simulink model "FAST"  (R2017b)
settings: Solver=FixedStepAuto  StartTime=0.0  StopTime=TMax  FixedStep=DT  RelTol=1e-3
values from neighbouring files (symbols this model uses):
  CertificationSettings = handles.CertificationSettings    [Certification.m]
  Control = handles.Control    [Certification.m]    (also in Linearization.m)
  dLP = ss(c2d(LP, Control.DT))    [ControllerDesign.m]
  dLP_IPC = ss(c2d(LP_IPC, Control.DT))    [ControllerDesign.m]
  dNotch = ss(c2d(Notch, Control.DT))    [ControllerDesign.m]
  Drivetrain = handles.Drivetrain    [Certification.m]    (also in Linearization.m)
  P_InitAngle = Control.Pitch.Max    [Certification.m]
  RPM_Init = 0    [Certification.m]
undefined symbols (not defined in the file or in its folder): AziPhase_offset_rev_1P, AziPhase_offset_rev_2P, DisableIPC_1P, DisableIPC_2P, DiscIntNeverNeededParam, OutList, strmatch, T_GenSpeedInit
libraries: simulink x5
(part 2 of 2)

== system FAST/Controller/IPC_Regulation/Forward Coleman Transformation 1P ==
  Azimuth : Inport
  My_1 : Inport  Port=2
  My_2 : Inport  Port=3
  My_3 : Inport  Port=4
  Add1 : Sum  Inputs=+++
  Add2 : Sum  Inputs=+++
  CosMy1 : Trigonometry  Operator=cos
  CosMy2 : Trigonometry  Operator=cos
  CosMy3 : Trigonometry  Operator=cos
  Gain : Gain  Gain=2/3
  Gain1 : Gain  Gain=2/3
  Product{1..6} (6 alike) : Product  RndMeth=Zero
  SinMy1 : Trigonometry
  SinMy2 : Trigonometry
  SinMy3 : Trigonometry
  Sum : Sum  Inputs=|++
  Sum1 : Sum  Inputs=++|
  nHarmonic1 : Gain
  nHarmonic2 : Gain
  phi : Constant  Value=2*pi/3
  M_tilt : Outport
  M_yaw : Outport  Port=2
  wires:
  nHarmonic2/1 -> Sum/2, CosMy1/1, SinMy1/1
  nHarmonic1/1 -> Sum1/2, Sum/1
  phi/1 -> nHarmonic1/1
  Azimuth/1 -> nHarmonic2/1
  CosMy1/1 -> Product1/2
  CosMy2/1 -> Product2/2
  SinMy1/1 -> Product4/2
  SinMy2/1 -> Product5/2
  Sum/1 -> Sum1/1, CosMy2/1, SinMy2/1
  My_1/1 -> Product4/1, Product1/1
  My_2/1 -> Product5/1, Product2/1
  Product1/1 -> Add1/1
  Product2/1 -> Add1/2
  Product4/1 -> Add2/1
  Product5/1 -> Add2/2
  Add1/1 -> Gain/1
  Add2/1 -> Gain1/1
  Sum1/1 -> SinMy3/1, CosMy3/1
  Product3/1 -> Add1/3
  My_3/1 -> Product6/1, Product3/1
  CosMy3/1 -> Product3/2
  SinMy3/1 -> Product6/2
  Product6/1 -> Add2/3
  Gain/1 -> M_tilt/1
  Gain1/1 -> M_yaw/1

== system FAST/Controller/IPC_Regulation/Forward Coleman Transformation 3P ==
  Azimuth : Inport
  My_1 : Inport  Port=2
  My_2 : Inport  Port=3
  My_3 : Inport  Port=4
  Add1 : Sum  Inputs=+++
  Add2 : Sum  Inputs=+++
  CosMy1 : Trigonometry  Operator=cos
  CosMy2 : Trigonometry  Operator=cos
  CosMy3 : Trigonometry  Operator=cos
  Gain : Gain  Gain=2/3
  Gain1 : Gain  Gain=2/3
  Product{1..6} (6 alike) : Product  RndMeth=Zero
  SinMy1 : Trigonometry
  SinMy2 : Trigonometry
  SinMy3 : Trigonometry
  Sum : Sum  Inputs=|++
  Sum1 : Sum  Inputs=++|
  nHarmonic : Gain  Gain=3
  nHarmonic1 : Gain  Gain=3
  phi : Constant  Value=2*pi/3
  M_tilt : Outport
  M_yaw : Outport  Port=2
  wires:
  nHarmonic1/1 -> SinMy1/1, CosMy1/1, Sum/2
  nHarmonic/1 -> Sum/1, Sum1/2
  Gain1/1 -> M_yaw/1
  Gain/1 -> M_tilt/1
  Product6/1 -> Add2/3
  SinMy3/1 -> Product6/2
  CosMy3/1 -> Product3/2
  My_3/1 -> Product3/1, Product6/1
  Product3/1 -> Add1/3
  Sum1/1 -> CosMy3/1, SinMy3/1
  Add2/1 -> Gain1/1
  Add1/1 -> Gain/1
  Product5/1 -> Add2/2
  Product4/1 -> Add2/1
  Product2/1 -> Add1/2
  Product1/1 -> Add1/1
  My_2/1 -> Product2/1, Product5/1
  My_1/1 -> Product1/1, Product4/1
  Sum/1 -> SinMy2/1, CosMy2/1, Sum1/1
  SinMy2/1 -> Product5/2
  SinMy1/1 -> Product4/2
  CosMy2/1 -> Product2/2
  CosMy1/1 -> Product1/2
  Azimuth/1 -> nHarmonic1/1
  phi/1 -> nHarmonic/1

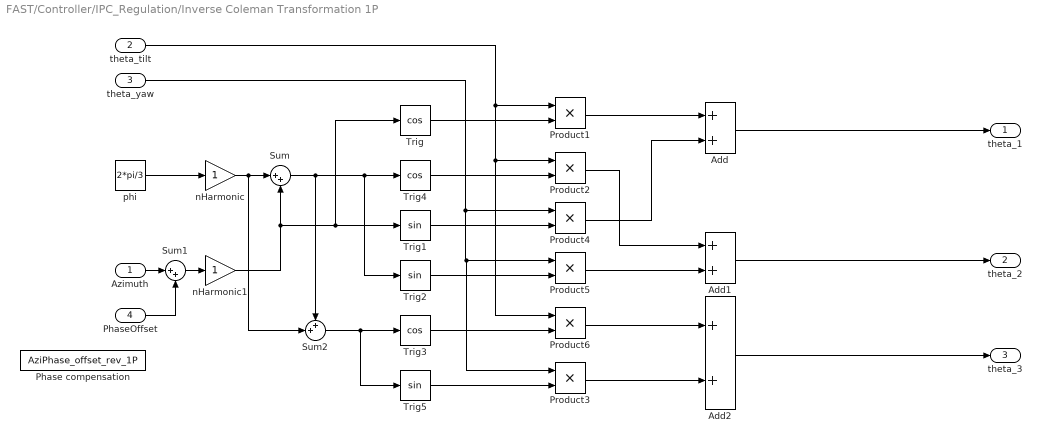
== system FAST/Controller/IPC_Regulation/Inverse Coleman Transformation 1P ==
  Azimuth : Inport
  theta_tilt : Inport  Port=2
  theta_yaw : Inport  Port=3
  PhaseOffset : Inport  Port=4
  Add : Sum
  Add1 : Sum
  Add2 : Sum
  Phase compensation : Constant  Value=AziPhase_offset_rev_1P
  Product{1..6} (6 alike) : Product  RndMeth=Zero
  Sum : Sum  Inputs=|++
  Sum1 : Sum  Inputs=|++
  Sum2 : Sum  Inputs=++|
  Trig : Trigonometry  Operator=cos
  Trig1 : Trigonometry
  Trig2 : Trigonometry
  Trig3 : Trigonometry  Operator=cos
  Trig4 : Trigonometry  Operator=cos
  Trig5 : Trigonometry
  nHarmonic : Gain
  nHarmonic1 : Gain
  phi : Constant  Value=2*pi/3
  theta_1 : Outport
  theta_2 : Outport  Port=2
  theta_3 : Outport  Port=3
  wires:
  Sum1/1 -> nHarmonic1/1
  Azimuth/1 -> Sum1/1
  nHarmonic/1 -> Sum/1, Sum2/2
  Add2/1 -> theta_3/1
  Add1/1 -> theta_2/1
  Add/1 -> theta_1/1
  Trig5/1 -> Product3/2
  Trig3/1 -> Product6/2
  Sum2/1 -> Trig3/1, Trig5/1
  Product3/1 -> Add2/2
  Product6/1 -> Add2/1
  PhaseOffset/1 -> Sum1/2
  Product5/1 -> Add1/2
  Product2/1 -> Add1/1
  Product1/1 -> Add/1
  Product4/1 -> Add/2
  theta_yaw/1 -> Product4/1, Product5/1, Product3/1
  theta_tilt/1 -> Product2/1, Product6/1, Product1/1
  Trig2/1 -> Product5/2
  Trig1/1 -> Product4/2
  Trig4/1 -> Product2/2
  Trig/1 -> Product1/2
  Sum/1 -> Trig2/1, Trig4/1, Sum2/1
  nHarmonic1/1 -> Sum/2, Trig1/1, Trig/1
  phi/1 -> nHarmonic/1

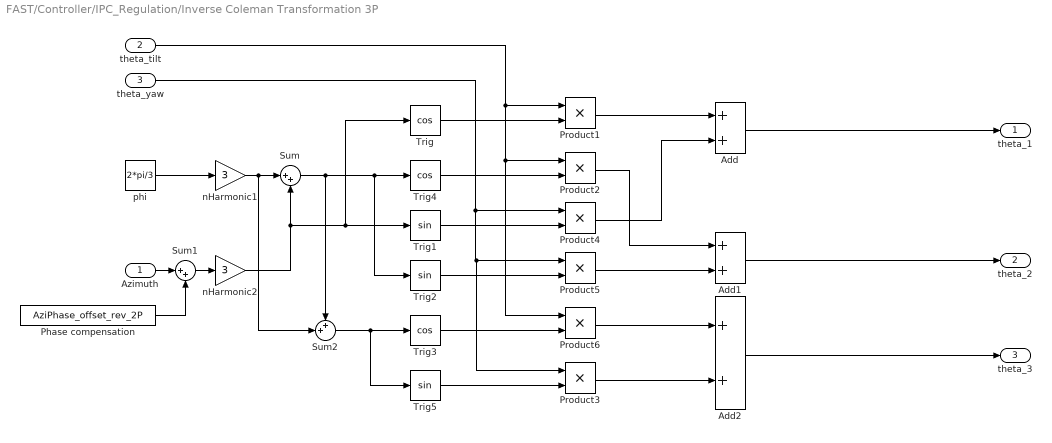
== system FAST/Controller/IPC_Regulation/Inverse Coleman Transformation 3P ==
  Azimuth : Inport
  theta_tilt : Inport  Port=2
  theta_yaw : Inport  Port=3
  Add : Sum
  Add1 : Sum
  Add2 : Sum
  Phase compensation : Constant  Value=AziPhase_offset_rev_2P
  Product{1..6} (6 alike) : Product  RndMeth=Zero
  Sum : Sum  Inputs=|++
  Sum1 : Sum  Inputs=|++
  Sum2 : Sum  Inputs=++|
  Trig : Trigonometry  Operator=cos
  Trig1 : Trigonometry
  Trig2 : Trigonometry
  Trig3 : Trigonometry  Operator=cos
  Trig4 : Trigonometry  Operator=cos
  Trig5 : Trigonometry
  nHarmonic1 : Gain  Gain=3
  nHarmonic2 : Gain  Gain=3
  phi : Constant  Value=2*pi/3
  theta_1 : Outport
  theta_2 : Outport  Port=2
  theta_3 : Outport  Port=3
  wires:
  nHarmonic2/1 -> Trig/1, Trig1/1, Sum/2
  Azimuth/1 -> Sum1/1
  nHarmonic1/1 -> Sum2/2, Sum/1
  phi/1 -> nHarmonic1/1
  Sum1/1 -> nHarmonic2/1
  Sum/1 -> Sum2/1, Trig4/1, Trig2/1
  Trig/1 -> Product1/2
  Trig4/1 -> Product2/2
  Trig1/1 -> Product4/2
  Trig2/1 -> Product5/2
  theta_tilt/1 -> Product1/1, Product6/1, Product2/1
  theta_yaw/1 -> Product3/1, Product5/1, Product4/1
  Product4/1 -> Add/2
  Product1/1 -> Add/1
  Product2/1 -> Add1/1
  Product5/1 -> Add1/2
  Phase compensation/1 -> Sum1/2
  Product6/1 -> Add2/1
  Product3/1 -> Add2/2
  Sum2/1 -> Trig5/1, Trig3/1
  Trig3/1 -> Product6/2
  Trig5/1 -> Product3/2
  Add/1 -> theta_1/1
  Add1/1 -> theta_2/1
  Add2/1 -> theta_3/1

== system FAST/Controller/Pitch Control/GainScheduler ==
  MeasuredPitch : Inport
  GainScheduled : Constant  Value=Control.Pitch.Scheduled
  GainScheduler_KpKi : MATLAB Function  TreatAsAtomicUnit=on
  KiGS : Lookup_n-D  NumberOfTableDimensions=1  BreakpointsForDimension1=Control.Pitch.ScheduledPitchAngles  Table=Control.Pitch.KiGS  ExtrapMethod=Clip  UseLastTableValue=on  InternalRulePriority=Speed  RndMeth=Simplest  InputSameDT=on
  KpGs : Lookup_n-D  NumberOfTableDimensions=1  BreakpointsForDimension1=Control.Pitch.ScheduledPitchAngles  Table=Control.Pitch.KpGS  ExtrapMethod=Clip  UseLastTableValue=on  InternalRulePriority=Speed  RndMeth=Simplest  InputSameDT=on
  KpKi : Constant  Value=[Control.Pitch.Kp Control.Pitch.Ki]
  Kp : Outport
  Ki : Outport  Port=2
  wires:
  MeasuredPitch/1 -> KiGS/1, KpGs/1
  GainScheduled/1 -> GainScheduler_KpKi/4(Scheduled)
  GainScheduler_KpKi/2(Ki_out) -> Ki/1
  KpKi/1 -> GainScheduler_KpKi/3(KpKi)
  KpGs/1 -> GainScheduler_KpKi/1(KpGS)
  KiGS/1 -> GainScheduler_KpKi/2(KiGS)
  GainScheduler_KpKi/1(Kp_out) -> Kp/1

== system FAST/Controller/Pitch Control/Lowpass Filter ==
  Input : Inport
  Discrete State-Space : DiscreteStateSpace  A=dLP.a  B=dLP.b  C=dLP.c  D=dLP.d  SampleTime=-1
  Output : Outport
  wires:
  Input/1 -> Discrete State-Space/1
  Discrete State-Space/1 -> Output/1

== system FAST/Controller/Torque Control/Low-pass filter ==
  Input : Inport
  Low-pass filter : DiscreteStateSpace  A=dLP.a  B=dLP.b  C=dLP.c  D=dLP.d  InitialCondition=T_GenSpeedInit*(pi/30)/dLP.c  SampleTime=-1
  Output : Outport
  wires:
  Input/1 -> Low-pass filter/1
  Low-pass filter/1 -> Output/1

== system FAST/Controller/Wind speed estimator_Gijs/Lowpass Filter ==
  Input : Inport
  Discrete State-Space : DiscreteStateSpace  A=dNotch.a  B=dNotch.b  C=dNotch.c  D=dNotch.d  SampleTime=-1
  Output : Outport
  wires:
  Discrete State-Space/1 -> Output/1
  Input/1 -> Discrete State-Space/1

== system FAST/Controller/Wind speed estimator_Sebas/Lowpass Filter ==
  Input : Inport
  Discrete State-Space : DiscreteStateSpace  A=dNotch.a  B=dNotch.b  C=dNotch.c  D=dNotch.d  SampleTime=-1
  Output : Outport
  wires:
  Input/1 -> Discrete State-Space/1
  Discrete State-Space/1 -> Output/1

== matlab function FAST/Controller/Rate Saturation Torque ==
  data: u input; MinSaturation input; y_out output; MaxSaturation input; DT input
function y_out = fcn(u, MinSaturation, MaxSaturation, DT)
persistent y

if isempty(y)
    y = u;
end

rate = (u-y)/DT;
rate = min(max(rate, MinSaturation), MaxSaturation);

y = y + rate*DT;
y_out = y;

== matlab function FAST/Controller/Rate Saturation Pitch ==
  data: u input; MinSaturation input; y_out output; MaxSaturation input; DT input
function y_out = fcn(u, MinSaturation, MaxSaturation, DT)
persistent y

if isempty(y)
    y = u;
end

rate = (u-y)/DT;
rate = min(max(rate, MinSaturation), MaxSaturation);

y = y + rate*DT;
y_out = y;

== matlab function FAST/Controller/Torque Control/TorqueController ==
  data: MeasuredTorque input; GeneratorTorqueDemand output; MeasuredGeneratorSpeed input; MeasuredPitch input; Control_Torque_OptGain input; omega_ABCD input size=[1 4]; P_StartupMode input; Torque_Demanded input; Pitch_Fine input; T_MinTorque input; KpKi_TorqueControl input; DT input
function GeneratorTorqueDemand  = TorqueController(MeasuredTorque, MeasuredGeneratorSpeed, MeasuredPitch, Control_Torque_OptGain, omega_ABCD, P_StartupMode, Torque_Demanded, Pitch_Fine, T_MinTorque, KpKi_TorqueControl, DT)
persistent Iterm

% Calculate generator torque setpoint according to the feedforward wind
% turbine control law T = K*\omega^2
GeneratorTorqueDemand = max(min(Control_Torque_OptGain*MeasuredGeneratorSpeed^2, Torque_Demanded), T_MinTorque);

% Calculate torques at beginning and end of CP_max operation
TorqueOmegaB = Control_Torque_OptGain*(omega_ABCD(2)*pi/30)^2;
TorqueOmegaC = Control_Torque_OptGain*(omega_ABCD(4)*pi/30)^2;

if isempty(Iterm)
    Iterm = TorqueOmegaC;
end

% Always perform PI-control on generator speed error
SpeedError = (omega_ABCD(4)*pi/30)-MeasuredGeneratorSpeed;
Pterm = KpKi_TorqueControl(1)*SpeedError;
Iterm = Iterm + KpKi_TorqueControl(2)*SpeedError*DT;
Iterm = min(max(Iterm, TorqueOmegaC), Torque_Demanded);
PIterm = Pterm + Iterm;
PIterm = min(max(PIterm, TorqueOmegaC), Torque_Demanded);

% Apply maximum demanded torque when pitch is 1 degree above fine-pitch and
% the wind turbine is not in start-up mode.
if MeasuredPitch > (Pitch_Fine + 1)*pi/180 && P_StartupMode == false
    GeneratorTorqueDemand = Torque_Demanded;
    Iterm = Torque_Demanded;
elseif MeasuredGeneratorSpeed < omega_ABCD(1)*pi/30
    GeneratorTorqueDemand = T_MinTorque;
elseif MeasuredGeneratorSpeed < omega_ABCD(2)*pi/30
    GeneratorTorqueDemand = (TorqueOmegaB - T_MinTorque)/((omega_ABCD(2) - omega_ABCD(1))*pi/30)*(MeasuredGeneratorSpeed - omega_ABCD(1)*pi/30) + T_MinTorque;
elseif (MeasuredGeneratorSpeed >= omega_ABCD(4)*pi/30) || (MeasuredTorque > TorqueOmegaC*1.001)
%     GeneratorTorqueDemand = (Torque_Demanded - TorqueOmegaC)/((omega_ABCD(4) - omega_ABCD(3))*pi/30)*(MeasuredGeneratorSpeed - omega_ABCD(3)*pi/30) + TorqueOmegaC;
    GeneratorTorqueDemand = PIterm;
end

== matlab function FAST/Controller/Pitch Control/PitchControl ==
  settings: updateMethod=DISCRETE  sampleTime=Control.DT
  data: GeneratorSpeedError input; GeneratorSpeed input; MeasuredTorque input; MeasuredPitch input; BladePitch output; KP input; KI input; MinMaxPitch input; MinMaxPitchRate input; DT input; P_InitAngle input; P_StartupPitch input; GearboxRatio input; P_StartUpSpeed input; P_StartupPitchRate input; omega_C input; Demanded_torque input; Clock input; P_LowRateModeOut output; Event input; EventTime input; dbg1 output; dbg2 output; dbg3 output
function [BladePitch, P_LowRateModeOut, dbg1, dbg2, dbg3]  = PitchControl(GeneratorSpeedError, GeneratorSpeed, MeasuredTorque, MeasuredPitch, KP, KI, MinMaxPitch, MinMaxPitchRate, DT, P_InitAngle, P_StartupPitch, GearboxRatio, P_StartUpSpeed, P_StartupPitchRate, omega_C, Demanded_torque, Clock, Event, EventTime)
persistent I_term PI_term_old P_LowRateMode P_LowRateMode_old

%Initialize all persistent variables
if isempty(I_term)
    I_term = (P_InitAngle*pi/180);
    PI_term_old = (P_InitAngle*pi/180);
    P_LowRateMode = true;
    P_LowRateMode_old = true; %Used to detect change from start-up/below-rated to above-rated operation mode
end

%Event handling part
if ((Event == 2 && Clock >= EventTime) || (Event == 5 && Clock >= EventTime)) %Grid loss, emergency shutdown
    P_LowRateMode = false;
    P_MinPitchSat = MinMaxPitch(2)*pi/180;
elseif (Event == 4 && Clock >= EventTime) % Normal shutdown
    P_LowRateMode = true;
    P_MinPitchSat = MinMaxPitch(2)*pi/180;
elseif Event == 7 || Event == 6 % Idling and parked mode
    P_MinPitchSat = MinMaxPitch(2)*pi/180;
elseif MeasuredTorque > Demanded_torque*0.999 % Above-rated operating mode
    P_LowRateMode = false;
    P_MinPitchSat = MinMaxPitch(2)*pi/180;
    if P_LowRateMode ~= P_LowRateMode_old % On switching event between below-rated to above rated, reinitialize the integral term to ensure smooth transition
        I_term = MeasuredPitch;
    end
elseif ((Event == 3) || (GeneratorSpeed < P_StartUpSpeed*GearboxRatio*(pi/30))) % Normal startup 
    if Event == 3 && Clock < EventTime % Time is lower then "Start at:"-event time
        P_LowRateMode = true;
        P_MinPitchSat = MinMaxPitch(2)*pi/180;
    elseif (Event == 3 && Clock >= EventTime) && (GeneratorSpeed < P_StartUpSpeed*GearboxRatio*(pi/30)) % Time is higher then "Start at:"-event time, but generator speed is lower than StartupSpeed
        P_LowRateMode = true;
        P_MinPitchSat = P_StartupPitch*pi/180;
    else % Time is higher then "Start at:"-event time, and generator speed is higer than StartupSpeed
        P_LowRateMode = true;
        P_MinPitchSat = MinMaxPitch(1)*pi/180;
    end
else
    P_MinPitchSat = MinMaxPitch(1)*pi/180;
end
 
% Pitch controller, KP and KI are constant or gain-scheduled, depending on
% input. Integral term is saturated, lower bound is variable and depends on
% event or operatinig mode.
P_term = KP*GeneratorSpeedError;
I_term = I_term + KI*GeneratorSpeedError*DT;
I_term = min(max(I_term, MinMaxPitch(1)*pi/180), P_MinPitchSat);

PI_term = P_term + I_term;
PI_term_sat = min(max(PI_term, MinMaxPitch(1)*pi/180), P_MinPitchSat);

% Calculate and limit pitch rate. Limit on rate is subject to event or
% operating mode.
PitchRate = (PI_term_sat - PI_term_old)/DT;
if P_LowRateMode
    PitchRate = min(max(PitchRate, -P_StartupPitchRate*pi/180), P_StartupPitchRate*pi/180);
else
    PitchRate = min(max(PitchRate, MinMaxPitchRate(1)*pi/180), MinMaxPitchRate(2)*pi/180);
end
BladePitch = PI_term_old + PitchRate*DT;

% Write variables to persistent variables and/or outputs
PI_term_old = BladePitch;
P_LowRateModeOut = P_LowRateMode;
P_LowRateMode_old = P_LowRateMode;

dbg1 = P_MinPitchSat;
dbg2 = 0;
dbg3 = 0;
end

== matlab function FAST/Controller/Pitch Control/GainScheduler/GainScheduler_KpKi ==
  data: KpGS input; KiGS input; Kp_out output; KpKi input; Scheduled input; Ki_out output
function [Kp_out, Ki_out] = fcn(KpGS, KiGS, KpKi, Scheduled)

if Scheduled > 0.5
    Kp_out = KpGS;
    Ki_out = KiGS;
else
    Kp_out = KpKi(1);
    Ki_out = KpKi(2);
end
